simulink model "PMSM_FOC_sensorless"  (R2026a)
settings: Solver=FixedStepDiscrete  StopTime=10  FixedStep=Ts  EnableMultiTasking=on
InitFcn:
  | ParameterInit
undefined symbols (not defined in the file): drive, FAKF, motor, Ts
libraries: simulink x10, mcbhdlcontrolslib x10, matrix_library x8, mcbcontrolslib x6, mcbpositiondecoderlib x3, mcbsensorlessestimatorlib x2, mcbeeMathTransformLib x2, slpidlib x2, sl_discontinuities x1, mcbplantlib x1, autolibpmsminterior x1, realtime_pacer_lib x1
(part 1 of 3)
settings Model: SimulationMode=accelerator  SnapshotBufferSize=100  Creator=xueji  LastModifiedBy=xuejf
settings DataIOCC: SaveFormat=StructureWithTime
settings OptimizationCC: ConditionallyExecuteInputs=off  UseDivisionForNetSlopeComputation=on  GainParamInheritBuiltInType=on  UseFloatMulNetSlope=on  StrengthReduction=on  NoFixptDivByZeroProtection=on  EfficientFloat2IntCast=on  OptimizationPriority=Speed  MultiThreadedLoops=on  AutoScheduleForLoops=on  UseRestrictQualifier=on
settings DebuggingCC: ParameterOverflowMsg=none  ParameterUnderflowMsg=error  ParameterPrecisionLossMsg=none
settings HardwareCC: ProdLargestAtomicInteger=Long  ProdLargestAtomicFloat=Double  ProdHWDeviceType=ARM Compatible->ARM Cortex  TargetBitPerPointer=64.0  TargetBitPerSizeT=64.0  TargetBitPerPtrDiffT=64.0  TargetLongLongMode=on  TargetIntDivRoundTo=Zero  TargetEndianess=LittleEndian  TargetWordSize=64.0  TargetHWDeviceType=MATLAB Host  ProdEqTarget=off
settings SFSimCC: SimTargetLang=C++
settings RTWCC: SystemTargetFile=ert.tlc  GenCodeOnly=on  Toolchain=GNU Tools for ARM Embedded Processors  BuildConfiguration=Faster Runs  DataTypeReplacement=CDataTypesFixedWidth  Description=Embedded Coder
settings CodeAppCC: CustomSymbolStrGlobalVar=rt$N$M  CustomSymbolStrType=$N$M  CustomSymbolStrFcn=$N$M$F  CustomSymbolStrMacro=$N$M  UseSimReservedNames=on
settings ERTTargetCC: ExtModeTransport=1.0  ExtModeMexFile=ext_serial_win32_comm  RootIOFormat=Structure reference  ERTFilePackagingFormat=Compact  IndentSize=4  MaxIdInt64=INT64_MAX  MinIdInt64=INT64_MIN  MaxIdUint64=UINT64_MAX  MaxIdInt32=INT32_MAX  MinIdInt32=INT32_MIN  MaxIdUint32=UINT32_MAX  MaxIdInt16=INT16_MAX  MinIdInt16=INT16_MIN  MaxIdUint16=UINT16_MAX  MaxIdInt8=INT8_MAX  MinIdInt8=INT8_MIN  MaxIdUint8=UINT8_MAX  DynamicArrayContainerType=coder::array  SupportAbsoluteTime=off  CodeInterfacePackaging=Reusable function  SupportComplex=off
settings SimscapeCC: SimscapeNominalValues="[{\"value\":\"1\",\"unit\":\"A\"},{\"value\":\"1\",\"unit\":\"bar\"},{\"value\":\"1\",\"unit\":\"cm^2\"},{\"value\":\"1\",\"unit\":\"cm^3/s\"},{\"value\":\"1\",\"unit\":\"kJ/kg\"},{\"value\":\"1\",\"unit\":\"kW\"},{\"value\":\"1\",\"unit\":\"l\"},{\"value\":\"1\",\"unit\":\"N\"},{\"value\":\"1\",\"unit\":\"N*m\"},{\"value\":\"1\",\"unit\":\"V\"}]"  SimscapeLogType=none  SimscapeLogDataHistory=5000.0

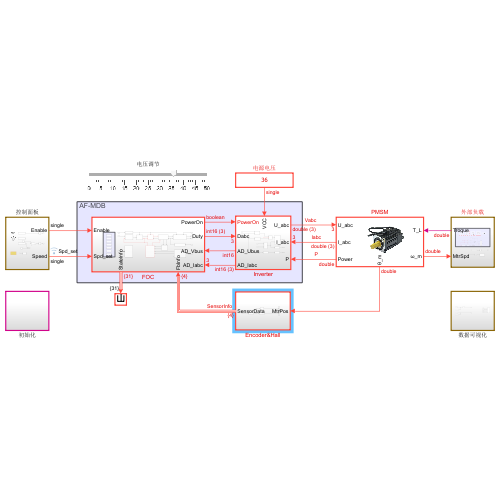
[thumbnail: Simulink's stored preview of the top-level diagram]
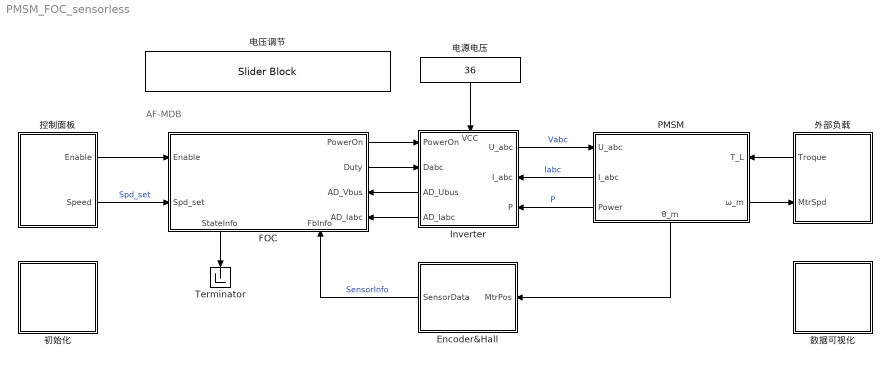
== system PMSM_FOC_sensorless ==
  note: AF-MDB
  Encoder&Hall : Subsystem
      settings: PortSchema="{\"entries\":[{\"content\":{\"sides\":[{\"content\":{\"connectorIds\":[\"Out1\"]},\"type\":\"ConnectorPlacement.EquallySpacedRectSide\",\"uuid\":\"8fa3dea7-ffc3-491e-9276-c955a36c6f18\"},{\"content\":{\"connectorIds\":[\"In1\"],\"side\":\"RIGHT\"},\"type\":\"ConnectorPlacement.EquallySpacedRectSide\",\"uuid\":\"8834e5d4-3827-462b-95b1-89ca8135bf93\"},{\"content\":{\"connectorIds\":[],\"side\":\"TOP\"},\"type\":\"ConnectorPlacement.EquallySpacedRectSide\",\"uuid\":\"076dd7d4-9aaa-4226-b42d-66fe25b6b28f\"}]},\"type\":\"ConnectorPlacement.EquallySpacedConnector\",\"uuid\":\"9a578460-81ff-4443-b5ec-3bd826764958\"}],\"packageUris\":[\"http://schema.mathworks.com/mf0/Connector/R2020b\"],\"version\":\"1.0\"}"
  FOC : Subsystem
      settings: PortSchema="{\"entries\":[{\"content\":{\"sides\":[{\"content\":{\"connectorIds\":[\"In1\",\"In2\"]},\"type\":\"ConnectorPlacement.EquallySpacedRectSide\",\"uuid\":\"46e73fc8-9e26-46f5-900f-d300c3d3ffa4\"},{\"content\":{\"connectorIds\":[\"Out1\",\"Out2\",\"In4\",\"In5\"],\"side\":\"RIGHT\"},\"type\":\"ConnectorPlacement.EquallySpacedRectSide\",\"uuid\":\"f8f13760-52ab-4821-8986-2e35fedfc95a\"},{\"content\":{\"side\":\"TOP\"},\"type\":\"ConnectorPlacement.EquallySpacedRectSide\",\"uuid\":\"3755d0d3-c979-48bd-b55d-3cbbf7594976\"},{\"content\":{\"connectorIds\":[\"Out3\",\"In3\"],\"side\":\"BOTTOM\"},\"type\":\"ConnectorPlacement.EquallySpacedRectSide\",\"uuid\":\"2c00eda5-e8e0-415c-bf0a-f2eb27cf355a\"}]},\"type\":\"ConnectorPlacement.EquallySpacedConnector\",\"uuid\":\"0d2281d8-e320-4044-ba1a-0a9e2c9cef92\"}],\"packageUris\":[\"http://schema.mathworks.com/mf0/Connector/R2020b\"],\"version\":\"1.0\"}"
  Inverter : Subsystem
      settings: PortSchema="{\"entries\":[{\"content\":{\"sides\":[{\"content\":{\"connectorIds\":[\"In1\",\"In2\",\"Out2\",\"Out3\"]},\"type\":\"ConnectorPlacement.EquallySpacedRectSide\",\"uuid\":\"edbc1bf3-6f5f-4012-892f-584587f9ac82\"},{\"content\":{\"connectorIds\":[\"Out1\",\"In4\",\"In5\"],\"side\":\"RIGHT\"},\"type\":\"ConnectorPlacement.EquallySpacedRectSide\",\"uuid\":\"6f51a7d6-6c28-4294-91cd-551043c21fcb\"},{\"content\":{\"connectorIds\":[\"In3\"],\"side\":\"TOP\"},\"type\":\"ConnectorPlacement.EquallySpacedRectSide\",\"uuid\":\"ca45aa73-ffa8-42f2-be70-f61dd7061c22\"}]},\"type\":\"ConnectorPlacement.EquallySpacedConnector\",\"uuid\":\"c09c89a4-9801-4f10-8b25-4ff06a898cdd\"}],\"packageUris\":[\"http://schema.mathworks.com/mf0/Connector/R2020b\"],\"version\":\"1.0\"}"
  PMSM : Subsystem
      settings: PortSchema="{\"entries\":[{\"content\":{\"sides\":[{\"content\":{\"connectorIds\":[\"In1\",\"Out3\",\"Out4\"]},\"type\":\"ConnectorPlacement.EquallySpacedRectSide\",\"uuid\":\"c2b23440-fc85-4d9c-858e-b988650f87d0\"},{\"content\":{\"connectorIds\":[\"In2\",\"Out1\"],\"side\":\"RIGHT\"},\"type\":\"ConnectorPlacement.EquallySpacedRectSide\",\"uuid\":\"6d28ba24-87ca-4dc4-bb5b-31bd216445dc\"},{\"content\":{\"side\":\"TOP\"},\"type\":\"ConnectorPlacement.EquallySpacedRectSide\",\"uuid\":\"4591baad-8ef3-475b-84da-7f88249a3560\"},{\"content\":{\"connectorIds\":[\"Out2\"],\"side\":\"BOTTOM\"},\"type\":\"ConnectorPlacement.EquallySpacedRectSide\",\"uuid\":\"01b968b1-c8c0-4355-9518-8898278f5093\"}]},\"type\":\"ConnectorPlacement.EquallySpacedConnector\",\"uuid\":\"f1130276-be58-456e-bfcb-28f536690efa\"}],\"packageUris\":[\"http://schema.mathworks.com/mf0/Connector/R2020b\"],\"version\":\"1.0\"}"
      mask Display: image('$imagefile'); % 使用工具条上的 "编辑图像" 进行更改。
  Terminator : Terminator
  初始化 : Subsystem
  外部负载 : Subsystem
      settings: PortSchema="{\"entries\":[{\"content\":{\"sides\":[{\"content\":{\"connectorIds\":[]},\"type\":\"ConnectorPlacement.EquallySpacedRectSide\",\"uuid\":\"5c626d5b-bf7f-42ce-ab58-2d542e2344bf\"},{\"content\":{\"connectorIds\":[\"Out1\",\"In1\"],\"side\":\"RIGHT\"},\"type\":\"ConnectorPlacement.EquallySpacedRectSide\",\"uuid\":\"d15cb2d3-f4cc-4d71-a0ed-13294ce13e05\"},{\"content\":{\"connectorIds\":[],\"side\":\"TOP\"},\"type\":\"ConnectorPlacement.EquallySpacedRectSide\",\"uuid\":\"7acbd73b-52e8-4e77-ba06-f51650d8c153\"}]},\"type\":\"ConnectorPlacement.EquallySpacedConnector\",\"uuid\":\"b6d8bd3c-2124-439b-8d25-1ae7167828cc\"}],\"packageUris\":[\"http://schema.mathworks.com/mf0/Connector/R2020b\"],\"version\":\"1.0\"}"
  控制面板 : Subsystem
  数据可视化 : Subsystem
  电压调节 : SliderBlock  LabelPosition=Hide  ScaleMax=50  TickInterval=5
  电源电压 : Constant  Value=36  OutDataTypeStr=single  SampleTime=Ts
  wires:
  Inverter/1(U_abc) -> PMSM/1(U_abc)  "Vabc"
  电源电压/1 -> Inverter/3(VCC)
  FOC/2(Duty) -> Inverter/2(Dabc)
  控制面板/1(Enable) -> FOC/1(Enable)
  控制面板/2(Speed) -> FOC/2(Spd_set)  "Spd_set"
  外部负载/1(Troque) -> PMSM/2(T_L)
  PMSM/1(ω_m) -> 外部负载/1(MtrSpd)
  PMSM/3(I_abc) -> Inverter/4(I_abc)  "Iabc"
  Inverter/2(AD_Ubus) -> FOC/4(AD_Vbus)
  FOC/3(StateInfo) -> Terminator/1
  FOC/1(PowerOn) -> Inverter/1(PowerOn)
  Inverter/3(AD_Iabc) -> FOC/5(AD_Iabc)
  PMSM/4(Power) -> Inverter/5(P)  "P"
  PMSM/2(θ_m) -> Encoder&Hall/1(MtrPos)
  Encoder&Hall/1(SensorData) -> FOC/3(FbInfo)  "SensorInfo"

== system PMSM_FOC_sensorless/Encoder&Hall ==
  MtrPos : Inport
  Bus Creator : BusCreator  Inputs=2
  Data Type Conversion3 : DataTypeConversion  OutDataTypeStr=single  SaturateOnIntegerOverflow=off  RndMeth=Floor
  编码器 : Subsystem
  霍尔传感器 : Subsystem
  SensorData : Outport
  wires:
  Bus Creator/1 -> SensorData/1
  编码器/1(编码值) -> Bus Creator/2  "Encoder"
  MtrPos/1 -> Data Type Conversion3/1
  Data Type Conversion3/1 -> 编码器/1(<MtrPos>), 霍尔传感器/1(MtrPos)  "MtrPos"
  霍尔传感器/1(Hall) -> Bus Creator/1  "Hall"

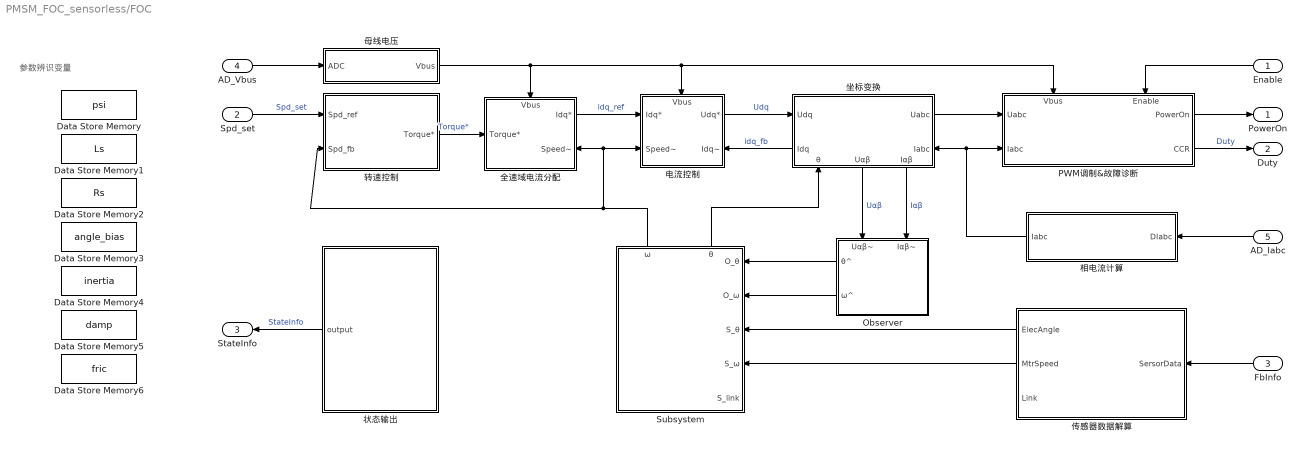
== system PMSM_FOC_sensorless/FOC ==
  note: 参数辨识变量
  Enable : Inport
  Spd_set : Inport  Port=2
  FbInfo : Inport  Port=3
  AD_Vbus : Inport  Port=4
  AD_Iabc : Inport  Port=5
  Data Store Memory : DataStoreMemory  DataStoreName=psi  WriteAfterWriteMsg=warning  ShowAdditionalParam=off
  Data Store Memory1 : DataStoreMemory  DataStoreName=Ls  WriteAfterWriteMsg=warning  ShowAdditionalParam=off
  Data Store Memory2 : DataStoreMemory  DataStoreName=Rs  WriteAfterWriteMsg=warning  ShowAdditionalParam=off
  Data Store Memory3 : DataStoreMemory  DataStoreName=angle_bias  WriteAfterWriteMsg=warning  ShowAdditionalParam=off  OutDataTypeStr=single
  Data Store Memory4 : DataStoreMemory  DataStoreName=inertia  WriteAfterWriteMsg=warning  ShowAdditionalParam=off  OutDataTypeStr=single
  Data Store Memory5 : DataStoreMemory  DataStoreName=damp  WriteAfterWriteMsg=warning  ShowAdditionalParam=off  OutDataTypeStr=single
  Data Store Memory6 : DataStoreMemory  DataStoreName=fric  WriteAfterWriteMsg=warning  ShowAdditionalParam=off  OutDataTypeStr=single
  Observer : Subsystem
      settings: MinAlgLoopOccurrences=on  PortSchema="{\"entries\":[{\"content\":{\"sides\":[{\"content\":{\"connectorIds\":[\"Out1\",\"Out2\"]},\"type\":\"ConnectorPlacement.EquallySpacedRectSide\",\"uuid\":\"e0bc5786-ce1d-4855-a3b5-736cd4452aa5\"},{\"content\":{\"side\":\"RIGHT\"},\"type\":\"ConnectorPlacement.EquallySpacedRectSide\",\"uuid\":\"2fd42ec2-cdfa-4ba6-bbae-150322a5d493\"},{\"content\":{\"connectorIds\":[\"In1\",\"In2\"],\"side\":\"TOP\"},\"type\":\"ConnectorPlacement.EquallySpacedRectSide\",\"uuid\":\"b90c8681-3a82-4d31-b956-3e10c61bd992\"}]},\"type\":\"ConnectorPlacement.EquallySpacedConnector\",\"uuid\":\"5605c3b5-9268-4421-a61a-19e31e78b2b2\"}],\"packageUris\":[\"http://schema.mathworks.com/mf0/Connector/R2020b\"],\"version\":\"1.0\"}"
  PWM调制&故障诊断 : Subsystem
      settings: PortSchema="{\"entries\":[{\"content\":{\"sides\":[{\"content\":{\"connectorIds\":[\"In1\",\"In2\"]},\"type\":\"ConnectorPlacement.EquallySpacedRectSide\",\"uuid\":\"492d6452-e717-42c4-995f-3faa38429cae\"},{\"content\":{\"connectorIds\":[\"Out1\",\"Out2\"],\"side\":\"RIGHT\"},\"type\":\"ConnectorPlacement.EquallySpacedRectSide\",\"uuid\":\"a45b9f70-76fb-43db-a233-80127821733d\"},{\"content\":{\"connectorIds\":[\"In3\",\"In4\"],\"side\":\"TOP\"},\"type\":\"ConnectorPlacement.EquallySpacedRectSide\",\"uuid\":\"87480e42-0fd9-4078-9596-9cf4a8d8a61b\"},{\"content\":{\"side\":\"BOTTOM\"},\"type\":\"ConnectorPlacement.EquallySpacedRectSide\",\"uuid\":\"e85548a5-948a-4384-9ce6-748091ec18d7\"}]},\"type\":\"ConnectorPlacement.EquallySpacedConnector\",\"uuid\":\"18d7a9be-c392-4737-8548-f782ad0f8f26\"}],\"packageUris\":[\"http://schema.mathworks.com/mf0/Connector/R2020b\"],\"version\":\"1.0\"}"
  Subsystem : Subsystem
      settings: PortSchema="{\"entries\":[{\"content\":{\"sides\":[{\"content\":{},\"type\":\"ConnectorPlacement.EquallySpacedRectSide\",\"uuid\":\"d4a4fcc6-9eab-45aa-b231-b7af833cd8c6\"},{\"content\":{\"connectorIds\":[\"In1\",\"In2\",\"In3\",\"In4\",\"In5\"],\"side\":\"RIGHT\"},\"type\":\"ConnectorPlacement.EquallySpacedRectSide\",\"uuid\":\"bf374db6-391b-4179-b18d-5bc8f845fc33\"},{\"content\":{\"connectorIds\":[\"Out1\",\"Out2\"],\"side\":\"TOP\"},\"type\":\"ConnectorPlacement.EquallySpacedRectSide\",\"uuid\":\"b7b6826e-7c33-41ba-b3c7-d16a7d7beb3a\"}]},\"type\":\"ConnectorPlacement.EquallySpacedConnector\",\"uuid\":\"61c6cbd8-a55e-4c51-8b84-52df934ee1be\"}],\"packageUris\":[\"http://schema.mathworks.com/mf0/Connector/R2020b\"],\"version\":\"1.0\"}"
  传感器数据解算 : Subsystem
  全速域电流分配 : Subsystem
      settings: PortSchema="{\"entries\":[{\"content\":{\"sides\":[{\"content\":{\"connectorIds\":[\"In1\"]},\"type\":\"ConnectorPlacement.EquallySpacedRectSide\",\"uuid\":\"55c1d0af-1e12-4135-aa70-ca0befd6bb29\"},{\"content\":{\"connectorIds\":[\"Out1\",\"In3\"],\"side\":\"RIGHT\"},\"type\":\"ConnectorPlacement.EquallySpacedRectSide\",\"uuid\":\"d5856c39-d2d9-42bf-88a6-12c62f6eb837\"},{\"content\":{\"connectorIds\":[\"In2\"],\"side\":\"TOP\"},\"type\":\"ConnectorPlacement.EquallySpacedRectSide\",\"uuid\":\"f04465a3-695d-494e-bf21-7b8ba0e1a298\"}]},\"type\":\"ConnectorPlacement.EquallySpacedConnector\",\"uuid\":\"e6412d78-9d8b-45ef-81b3-23a4fb87ae10\"}],\"packageUris\":[\"http://schema.mathworks.com/mf0/Connector/R2020b\"],\"version\":\"1.0\"}"
  坐标变换 : Subsystem
      settings: PortSchema="{\"entries\":[{\"content\":{\"sides\":[{\"content\":{\"connectorIds\":[\"In1\",\"Out4\"]},\"type\":\"ConnectorPlacement.EquallySpacedRectSide\",\"uuid\":\"19423b74-9855-4da1-a32f-fc09d117de38\"},{\"content\":{\"connectorIds\":[\"Out1\",\"In3\"],\"side\":\"RIGHT\"},\"type\":\"ConnectorPlacement.EquallySpacedRectSide\",\"uuid\":\"45d897d7-b2dc-4681-bc4b-90a4bd929118\"},{\"content\":{\"connectorIds\":[],\"side\":\"TOP\"},\"type\":\"ConnectorPlacement.EquallySpacedRectSide\",\"uuid\":\"59354a96-0169-49af-a302-86e785c620a3\"},{\"content\":{\"connectorIds\":[\"In2\",\"Out2\",\"Out3\"],\"side\":\"BOTTOM\"},\"type\":\"ConnectorPlacement.EquallySpacedRectSide\",\"uuid\":\"fb332ee8-d153-4216-8303-19cfa3862110\"}]},\"type\":\"ConnectorPlacement.EquallySpacedConnector\",\"uuid\":\"5f6d72a6-e6b8-48f2-bb88-1ad3720f15b2\"}],\"packageUris\":[\"http://schema.mathworks.com/mf0/Connector/R2020b\"],\"version\":\"1.0\"}"
  母线电压 : Subsystem
  状态输出 : Subsystem
      settings: PortSchema="{\"entries\":[{\"content\":{\"sides\":[{\"content\":{\"connectorIds\":[\"Out1\"]},\"type\":\"ConnectorPlacement.EquallySpacedRectSide\",\"uuid\":\"5ecb5947-9baa-4bfe-8641-96ff20667d62\"},{\"content\":{\"side\":\"RIGHT\"},\"type\":\"ConnectorPlacement.EquallySpacedRectSide\",\"uuid\":\"3d186154-f081-4d30-a108-1a942147f536\"},{\"content\":{\"side\":\"TOP\"},\"type\":\"ConnectorPlacement.EquallySpacedRectSide\",\"uuid\":\"5aa511f5-28fe-4d78-8a7e-f2efec5693a1\"}]},\"type\":\"ConnectorPlacement.EquallySpacedConnector\",\"uuid\":\"ee06c015-bb25-435b-b725-56d91e20a522\"}],\"packageUris\":[\"http://schema.mathworks.com/mf0/Connector/R2020b\"],\"version\":\"1.0\"}"
  电流控制 : Subsystem
      settings: PortSchema="{\"entries\":[{\"content\":{\"sides\":[{\"content\":{\"connectorIds\":[\"In1\",\"In2\"]},\"type\":\"ConnectorPlacement.EquallySpacedRectSide\",\"uuid\":\"bf76b923-f33f-405a-8981-aa5371d2085f\"},{\"content\":{\"connectorIds\":[\"Out1\",\"In4\"],\"side\":\"RIGHT\"},\"type\":\"ConnectorPlacement.EquallySpacedRectSide\",\"uuid\":\"e7d4bdbe-138f-4605-8031-f7f1fbb983cf\"},{\"content\":{\"connectorIds\":[\"In3\"],\"side\":\"TOP\"},\"type\":\"ConnectorPlacement.EquallySpacedRectSide\",\"uuid\":\"9cdf7367-4fd9-4634-a6c3-b049cc73c34c\"},{\"content\":{\"side\":\"BOTTOM\"},\"type\":\"ConnectorPlacement.EquallySpacedRectSide\",\"uuid\":\"aba65895-d8a9-40f0-9a72-aa89d29f659a\"}]},\"type\":\"ConnectorPlacement.EquallySpacedConnector\",\"uuid\":\"3c2b3690-9a24-4e84-8e12-40b94ce0a856\"}],\"packageUris\":[\"http://schema.mathworks.com/mf0/Connector/R2020b\"],\"version\":\"1.0\"}"
  相电流计算 : Subsystem
  转速控制 : Subsystem
  PowerOn : Outport
  Duty : Outport  Port=2
  StateInfo : Outport  Port=3
  wires:
  PWM调制&故障诊断/2(CCR) -> Duty/1  "Duty"
  坐标变换/4(Idq) -> 电流控制/4(Idq~)  "idq_fb"
  电流控制/1(Udq*) -> 坐标变换/1(Udq)  "Udq"
  坐标变换/1(Uabc) -> PWM调制&故障诊断/1(Uabc)
  Enable/1 -> PWM调制&故障诊断/4(Enable)
  坐标变换/2(Uαβ) -> Observer/1(Uαβ~)  "Uαβ"
  坐标变换/3(Iαβ) -> Observer/2(Iαβ~)  "Iαβ"
  Spd_set/1 -> 转速控制/1(Spd_ref)  "Spd_set"
  转速控制/1(Torque*) -> 全速域电流分配/1(Torque*)  "Torque*"
  全速域电流分配/1(Idq*) -> 电流控制/1(Idq*)  "idq_ref"
  相电流计算/1(Iabc) -> 坐标变换/3(Iabc), PWM调制&故障诊断/2(Iabc)
  FbInfo/1 -> 传感器数据解算/1(SersorData)
  状态输出/1(output) -> StateInfo/1  "StateInfo"
  PWM调制&故障诊断/1(PowerOn) -> PowerOn/1
  AD_Iabc/1 -> 相电流计算/1(DIabc)
  母线电压/1(Vbus) -> PWM调制&故障诊断/3(Vbus), 电流控制/3(Vbus), 全速域电流分配/2(Vbus)
  AD_Vbus/1 -> 母线电压/1(ADC)
  传感器数据解算/2(MtrSpeed) -> Subsystem/4(S_ω)
  传感器数据解算/1(ElecAngle) -> Subsystem/3(S_θ)
  Subsystem/1(ω) -> 电流控制/2(Speed~), 全速域电流分配/3(Speed~), 转速控制/2(Spd_fb)
  Observer/1(θ^) -> Subsystem/1(O_θ)
  Subsystem/2(θ) -> 坐标变换/2(θ)
  Observer/2(ω^) -> Subsystem/2(O_ω)

== system PMSM_FOC_sensorless/Inverter ==
  PowerOn : Inport
  Dabc : Inport  Port=2
  VCC : Inport  Port=3
  I_abc : Inport  Port=4
  P : Inport  Port=5
  AD转换 : Subsystem
  Data Type Conversion1 : DataTypeConversion  OutDataTypeStr=single  SaturateOnIntegerOverflow=off  RndMeth=Floor
  Switch : Switch  Criteria=u2 > Threshold  SaturateOnIntegerOverflow=off  InputSameDT=off
  模拟MOS管截至状态 : Subsystem  TreatAsAtomicUnit=on
  正常PWM调制 : Subsystem  TreatAsAtomicUnit=on
  母线压降 : Subsystem
  母线电压采样 : Subsystem
  逆变器 : mcbplantlib/Average-Value Inverter
  采样芯片 : Subsystem
  U_abc : Outport
  AD_Ubus : Outport  Port=2
  AD_Iabc : Outport  Port=3
  wires:
  逆变器/1 -> U_abc/1
  PowerOn/1 -> Switch/2
  模拟MOS管截至状态/1(Out1) -> Switch/3
  正常PWM调制/1(Out1) -> Switch/1
  Switch/1 -> 逆变器/1
  Dabc/1 -> 正常PWM调制/1(Dabc)
  Data Type Conversion1/1 -> 采样芯片/1(Iabc)  "Iabc"
  I_abc/1 -> Data Type Conversion1/1, 模拟MOS管截至状态/1(Iabc), 正常PWM调制/2(Iabc)
  AD转换/1(digital) -> AD_Iabc/1  "ADC_Iabc"
  采样芯片/1(Isabc) -> AD转换/1(analog)
  母线电压采样/1(AD_Ubus) -> AD_Ubus/1
  P/1 -> 母线压降/2(P)
  母线压降/1(U_bus) -> 母线电压采样/1(U_bus), 逆变器/2
  VCC/1 -> 母线压降/1(VCC)

== system PMSM_FOC_sensorless/PMSM ==
  U_abc : Inport
  T_L : Inport  Port=2
  Bus Selector : BusSelector  OutputSignals=PwrInfo.PwrTrnsfrd.PwrBus,MtrPos
  Interior PMSM : autolibpmsminterior/Interior PMSM  port_config=Torque  sim_type=Discrete  Ts=Ts  FilePath=interiorpmsm_motordata.m  P=motor.P  Rs=motor.Rs  Ldq=[motor.Ls motor.Ls]  KConstText=Back-emf constant (Ke):  lambda_pm=0.1194  Ke=motor.Ke  mechanical=[motor.J, motor.damp, motor.fric]  idq0=[0 0]  theta_init=motor.angle_init  omega_init=0  KConst=motor.Ke  lambda_pm_calc=0.010526  Kt=1.323  RefBlkName='autolibpmsminterior/Interior PMSM'  aMode=1
      settings: LibrarySourceBlock=autolibemachines/Interior PMSM
  Mechanical to Electrical Position : mcbpositiondecoderlib/Mechanical to Electrical Position  PolePairsInputType=Specify via dialog  NrPP=motor.P  selectedRange=Radians  MechOfstInputType=Specify via dialog  mechOffsetIn=0  maxAngleIn=2*pi  InputDataType=single  VariantSelect=floating-point
      settings: LibrarySourceBlock=mcblib/Sensor Decoders/Mechanical to Electrical Position
  Subsystem2 : Subsystem
  ω_m : Outport
  θ_m : Outport  Port=2
  I_abc : Outport  Port=3
  Power : Outport  Port=4
  tag scope: Real_Iabc=global, Real_LdTrq=global, Real_MotorInfo=global, Real_MtrSpd=global, Real_Theat_e=global, Real_Theat_m=global, Real_Vabc=global
  wires:
  T_L/1 -> [Real_LdTrq], Interior PMSM/1
  Interior PMSM/3 -> [Real_MtrSpd], ω_m/1  "ω_m"
  Interior PMSM/2 -> [Real_Iabc], I_abc/1
  Interior PMSM/1 -> [Real_MotorInfo], Bus Selector/1  "MotorInfo"
  U_abc/1 -> [Real_Vabc], Interior PMSM/2
  Bus Selector/2 -> Mechanical to Electrical Position/1, [Real_Theat_m], θ_m/1  "<MtrPos>"
  Bus Selector/1 -> Power/1  "<PwrBus>"
  Mechanical to Electrical Position/1 -> Subsystem2/1(0-2pi)
  Subsystem2/1(-pi-pi) -> [Real_Theat_e]  "θ_e"

== system PMSM_FOC_sensorless/初始化 ==

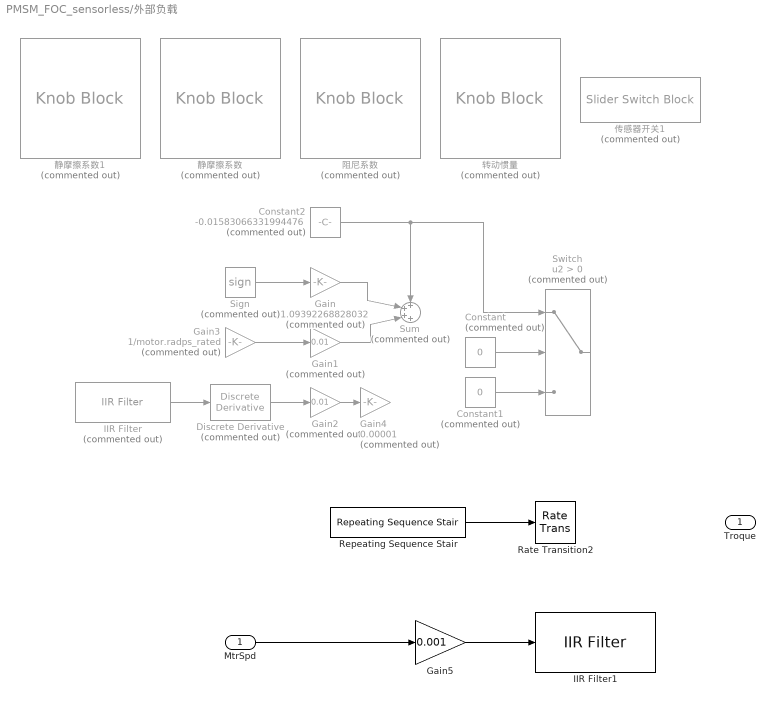
== system PMSM_FOC_sensorless/外部负载 ==
  MtrSpd : Inport
  Constant : Constant  Commented=on  Value=0
  Constant1 : Constant  Commented=on  Value=0
  Constant2 : Constant  Commented=on  Value=-0.01583066331994476
  Discrete Derivative : simulink/Discrete/Discrete Derivative  Commented=on  gainval=1.0  ICPrevScaledInput=0.0  OutMin=[]  OutMax=[]  OutDataType=fixdt(1, 16)  OutScaling=2^-10  DoSatur=off
  Gain : Gain  Commented=on  Gain=1.09392268828032
  Gain1 : Gain  Commented=on  Gain=0.01
  Gain2 : Gain  Commented=on  Gain=0.01
  Gain3 : Gain  Commented=on  Gain=1/motor.radps_rated
  Gain4 : Gain  Commented=on  Gain=0.00001
  Gain5 : Gain  Gain=0.001
  IIR Filter : mcbcontrolslib/IIR Filter  Commented=on  VariantControl=Low Pass Filter  VariantSelect=Low-pass  FilterConstantInputType=Specify via dialog  Filter_constant=0.1  advancedSettings=off  Ts=50e-6  cutOff_freq=353.6777
      settings: LibrarySourceBlock=mcbhdllib/Signal Management/IIR Filter
  IIR Filter1 : mcbhdlcontrolslib/IIR Filter  VariantControl=Low Pass Filter  VariantSelect=Low-pass  FilterConstantInputType=Specify via dialog  Filter_constant=0.01  advancedSettings=off  Ts=50e-6  cutOff_freq=32.1525
  Rate Transition2 : RateTransition  OutPortSampleTime=Ts
  Repeating Sequence Stair : simulink/Sources/Repeating Sequence Stair  OutValues=0.3*[0 0 0 motor.T_rated motor.T_rated motor.T_rated 0 0 0].'  tsamp=0.5  OutMin=[]  OutMax=[]  OutDataTypeStr=double  OutputDataTypeScalingMode=double  OutDataType=fixdt(0,8)  ConRadixGroup=Best Precision: Vector-wise  OutScaling=2^-12
  Sign : Signum  Commented=on
  Sum : Sum  Commented=on  Inputs=++++
  Switch : Switch  Commented=on  Criteria=u2 > Threshold  SaturateOnIntegerOverflow=off  InputSameDT=off
  传感器开关1 : SliderSwitchBlock  Commented=on
  转动惯量 : KnobBlock  Commented=on  ScaleMin=0.01  ScaleType=Log
  阻尼系数 : KnobBlock  Commented=on  ScaleMin=0.01  ScaleType=Log
  静摩擦系数 : KnobBlock  Commented=on  ScaleMin=0.01  ScaleType=Log
  静摩擦系数1 : KnobBlock  Commented=on  ScaleMin=-1  ScaleMax=1
  Troque : Outport
  wires:
  ? -> Sign/1, IIR Filter/1, Gain3/1
  Sign/1 -> Gain/1
  Gain/1 -> Sum/2
  Constant2/1 -> Switch/1, Sum/1
  Constant/1 -> Switch/2
  Constant1/1 -> Switch/3
  Discrete Derivative/1 -> Gain2/1
  Gain1/1 -> Sum/3
  Gain3/1 -> Gain1/1
  Gain2/1 -> Gain4/1
  IIR Filter/1 -> Discrete Derivative/1
  Repeating Sequence Stair/1 -> Rate Transition2/1
  MtrSpd/1 -> Gain5/1
  Gain5/1 -> IIR Filter1/1

== system PMSM_FOC_sensorless/控制面板 ==
  Clock : Clock
  Constant3 : Constant  OutDataTypeStr=single  SampleTime=Ts
  Gain3 : Gain  Gain=motor.radps_rated  OutDataTypeStr=single
  Knob : KnobBlock  ScaleMin=-1  ScaleMax=1
  MATLAB Function : MATLAB Function  TreatAsAtomicUnit=on
  Product : Product
  Rate Transition2 : RateTransition  OutPortSampleTime=Ts
  Rate Transition3 : RateTransition  OutPortSampleTime=Ts
  Real-Time Pacer : realtime_pacer_lib/Real-Time Pacer  Commented=on  simTimePerRealTime=0.1
      settings: SourceProductName=Real-Time Pacer
  Repeating Sequence Stair1 : simulink/Sources/Repeating Sequence Stair  OutValues=[0.05 -0.05 -1 1]  tsamp=0.5  OutMin=[]  OutMax=[]  OutDataTypeStr=double  OutputDataTypeScalingMode=double  OutDataType=fixdt(0,8)  ConRadixGroup=Best Precision: Vector-wise  OutScaling=2^-12
  Sine Wave : Sin  Amplitude=0.2  Bias=0.2  Frequency=2*pi  Phase=-pi/2  SampleTime=Ts
  Step : Step  SampleTime=0
  传感器开关 : SliderSwitchBlock
  可调 : Constant  Value=0.5764853922526041  OutDataTypeStr=single  SampleTime=Ts
  Enable : Outport
  Speed : Outport  Port=2
  wires:
  Gain3/1 -> Rate Transition2/1
  Constant3/1 -> Rate Transition3/1
  Rate Transition2/1 -> Speed/1
  Rate Transition3/1 -> Enable/1
  Sine Wave/1 -> Product/1
  Step/1 -> Product/2
  Repeating Sequence Stair1/1 -> Gain3/1
  Clock/1 -> MATLAB Function/1(t)

== system PMSM_FOC_sensorless/数据可视化 ==
  Sum : Sum  Inputs=|+-
  Sum1 : Sum  Inputs=|+-
  Terminator : Terminator
  Terminator1 : Terminator
  angle limit2 : Subsystem
  卡尔曼过程可视化 : Subsystem  mask{en=0, plot_freq=2000, buff_len=64, range=30}
      mask prompts: en "使能"; plot_freq "绘图频率"; buff_len "轨迹长度"; range "坐标范围"
      mask DialogControl DescGroupVar Prompt: 描述
      mask DialogControl DescTextVar Prompt: 卡尔曼观测器数据可视化
      mask DialogControl ParameterGroupVar Prompt: 参数
  wires:
  [x] -> 卡尔曼过程可视化/5(x_k)
  [x_1] -> 卡尔曼过程可视化/1(x_k|k-1)
  [P_1] -> 卡尔曼过程可视化/2(P_k|k-1)
  [z] -> 卡尔曼过程可视化/3(z_k)
  [R] -> 卡尔曼过程可视化/4(R)
  [P] -> 卡尔曼过程可视化/6(P_k)
  Sum/1 -> angle limit2/1(In)
  [Real_MtrSpd] -> Sum1/1
  angle limit2/1(Out) -> Terminator/1  "err_θ"
  Sum1/1 -> Terminator1/1  "err_ω"
  [Real_Theat_e] -> Sum/1
  [Observer_Speed_m] -> Sum1/2
  [Observer_Angle_e] -> Sum/2

== system PMSM_FOC_sensorless/Encoder&Hall/编码器 ==
  <MtrPos> : Inport
  Constant1 : Constant  Value=motor.ENC_CNT  OutDataTypeStr=int16
  Gain1 : Gain  Gain=motor.ENC_CNT/(2*pi)  OutDataTypeStr=int16
  Mod : Math  Operator=mod
  Sum : Sum  Inputs=|+-
  初始角度 : Constant  Value=motor.angle_init  OutDataTypeStr=single
  编码值 : Outport
  wires:
  <MtrPos>/1 -> Sum/1
  Sum/1 -> Gain1/1
  初始角度/1 -> Sum/2
  Constant1/1 -> Mod/2
  Gain1/1 -> Mod/1
  Mod/1 -> 编码值/1

== system PMSM_FOC_sensorless/Encoder&Hall/霍尔传感器 ==
  MtrPos : Inport
  Constant18 : Constant  Value=[1,0,1]  OutDataTypeStr=int8
  Constant19 : Constant  Value=[1,0,0]  OutDataTypeStr=int8
  Constant20 : Constant  Value=[1,1,0]  OutDataTypeStr=int8
  Constant21 : Constant  Value=[0,1,0]  OutDataTypeStr=int8
  Constant22 : Constant  Value=[0,1,1]  OutDataTypeStr=int8
  Constant23 : Constant  Value=[0,0,1]  OutDataTypeStr=int8
  Multiport Switch3 : MultiPortSwitch  DataPortOrder=Zero-based contiguous  Inputs=6  zeroidx=on  SaturateOnIntegerOverflow=off  InputSameDT=off
  Subsystem : Subsystem
  Hall : Outport
  wires:
  MtrPos/1 -> Subsystem/1(MtrPos)
  Subsystem/1(Phase) -> Multiport Switch3/1
  Multiport Switch3/1 -> Hall/1
  Constant18/1 -> Multiport Switch3/2
  Constant19/1 -> Multiport Switch3/3
  Constant20/1 -> Multiport Switch3/4
  Constant21/1 -> Multiport Switch3/5
  Constant22/1 -> Multiport Switch3/6
  Constant23/1 -> Multiport Switch3/7

== system PMSM_FOC_sensorless/FOC/Observer ==
  Uαβ~ : Inport
  Iαβ~ : Inport  Port=2
  AKF : Subsystem
  Demux : Demux  Outputs=2
  位置提取 : Subsystem
  对比观测器 : Subsystem  Commented=on
  角度转换 : Subsystem
  计算转子反电动势 : Subsystem
  转矩计算 : Subsystem
  θ^ : Outport
  ω^ : Outport  Port=2
  tag scope: Observer_Angle_e=global, Observer_Speed_m=global
  wires:
  Demux/1 -> ω^/1, [Observer_Speed_m]
  角度转换/1(sincos) -> 转矩计算/1(θ_sincos), 位置提取/2(θ_sincos)
  Uαβ~/1 -> 计算转子反电动势/2(Uαβ), 对比观测器/1(u)
  计算转子反电动势/1(Eαβ) -> 位置提取/1(Eαβ)  "E_αβ"
  Iαβ~/1 -> 计算转子反电动势/1(Iαβ), 转矩计算/2(I_αβ), 对比观测器/2(i)
  转矩计算/1(T) -> AKF/1(u_k)  "T"
  位置提取/1(ωθ) -> AKF/2(z_k)  "ωθ~"
  AKF/1(x_k) -> Demux/1
  Demux/2 -> [Observer_Angle_e], θ^/1, 角度转换/1(θ)

== system PMSM_FOC_sensorless/FOC/PWM调制&故障诊断 ==
  Uabc : Inport
  Iabc : Inport  Port=2
  Vbus : Inport  Port=3
  Enable : Inport  Port=4
  Constant : Constant  Value=0.5  OutDataTypeStr=single
  Divide : Product  Inputs=*/
  Gain1 : Gain  Gain=drive.dead_time/drive.T_PWM  OutDataTypeStr=single
  Gain3 : Gain  Gain=drive.CNT_PWM  OutDataTypeStr=int16
  NOT : Logic  Operator=NOT  IconShape=distinctive  AllPortsSameDT=off  OutDataTypeStr=boolean
  NOT1 : Logic  IconShape=distinctive  AllPortsSameDT=off  OutDataTypeStr=boolean
  Sign : Signum
  Sum : Sum  Inputs=+++
  故障诊断 : Subsystem
  限幅1 : Saturate  UpperLimit=drive.CNT_PWM*0.99  LowerLimit=drive.CNT_PWM*0.01
  PowerOn : Outport
  CCR : Outport  Port=2
  tag scope: U_bus=global
  wires:
  Divide/1 -> Sum/2  "Duty"
  Uabc/1 -> Divide/1
  限幅1/1 -> CCR/1
  Sign/1 -> Gain1/1
  Iabc/1 -> 故障诊断/1(I_abc), Sign/1
  Gain1/1 -> Sum/1
  NOT/1 -> NOT1/1
  Enable/1 -> NOT1/2
  故障诊断/1(Err_code) -> NOT/1
  NOT1/1 -> PowerOn/1
  Constant/1 -> Sum/3
  Sum/1 -> Gain3/1
  Vbus/1 -> [U_bus], Divide/2, 故障诊断/2(U_bus)
  Gain3/1 -> 限幅1/1

== system PMSM_FOC_sensorless/FOC/Subsystem ==
  O_θ : Inport
  O_ω : Inport  Port=2
  S_θ : Inport  Port=3
  S_ω : Inport  Port=4
  S_link : Inport  Port=5
  Switch : Switch  Criteria=u2 > Threshold  SaturateOnIntegerOverflow=off  InputSameDT=off
  Switch1 : Switch  Criteria=u2 > Threshold  SaturateOnIntegerOverflow=off  InputSameDT=off
  ω : Outport
  θ : Outport  Port=2
  wires:
  O_ω/1 -> Switch1/3
  S_θ/1 -> Switch/1
  O_θ/1 -> Switch/3
  S_ω/1 -> Switch1/1
  S_link/1 -> Switch1/2, Switch/2
  Switch/1 -> θ/1
  Switch1/1 -> ω/1

== system PMSM_FOC_sensorless/FOC/传感器数据解算 ==
  SersorData : Inport
  Bus Selector2 : BusSelector  OutputSignals=Hall,Encoder
  Terminator : Terminator
  角度计算 : Subsystem
  转速计算 : Subsystem
  ElecAngle : Outport
  MtrSpeed : Outport  Port=2
  Link : Outport  Port=3
  tag scope: Sensor_Angle_e=global, Sensor_Speed_m=global
  wires:
  SersorData/1 -> Bus Selector2/1
  角度计算/1(MtrPos) -> Terminator/1
  转速计算/1(MtrSpeed) -> [Sensor_Speed_m], MtrSpeed/1
  Bus Selector2/2 -> 转速计算/1(Encoder), 角度计算/2(Encoder)  "<Encoder>"
  Bus Selector2/1 -> 角度计算/1(Hall)  "<Hall>"
  角度计算/2(ElecAngle) -> [Sensor_Angle_e], ElecAngle/1
  角度计算/3(Link) -> Link/1

== system PMSM_FOC_sensorless/FOC/全速域电流分配 ==
  Torque* : Inport
  Vbus : Inport  Port=2
  Speed~ : Inport  Port=3
  Constant1 : Constant  Value=motor.I_max  OutDataTypeStr=single
  Gain : Gain  Gain=1/motor.Kt
  Gain2 : Gain  Gain=-1
  IIR Filter1 : mcbhdlcontrolslib/IIR Filter  VariantControl=Low Pass Filter  VariantSelect=Low-pass  FilterConstantInputType=Specify via dialog  Filter_constant=0.1  advancedSettings=off  Ts=50e-6  cutOff_freq=353.6777
  MJPA : Subsystem
  Math Function : Math  Operator=square
  Math Function1 : Math  Operator=square
  Mux1 : Mux  Inputs=2
  Saturation Dynamic : sl_discontinuities/Saturation Dynamic  OutMin=[]  OutMax=[]  OutDataTypeStr=single  OutDataType=fixdt(1, 16)  OutScaling=2^-10  DoSatur=off
  Sqrt : Sqrt
  Sum1 : Sum  Inputs=-+|
  Idq* : Outport
  tag scope: Speed_m=global
  wires:
  Saturation Dynamic/1 -> Mux1/2
  Mux1/1 -> IIR Filter1/1
  Torque*/1 -> Gain/1
  Speed~/1 -> MJPA/2(ω_m), [Speed_m]
  Constant1/1 -> Math Function1/1
  Math Function/1 -> Sum1/1
  Sum1/1 -> Sqrt/1
  Sqrt/1 -> Gain2/1, Saturation Dynamic/1
  Gain2/1 -> Saturation Dynamic/3
  Vbus/1 -> MJPA/1(Vbus)
  MJPA/1(i*_d) -> Math Function/1, Mux1/1
  Math Function1/1 -> Sum1/2
  IIR Filter1/1 -> Idq*/1
  Gain/1 -> Saturation Dynamic/2

== system PMSM_FOC_sensorless/FOC/坐标变换 ==
  Udq : Inport
  θ : Inport  Port=2
  Iabc : Inport  Port=3
  Subsystem11 : Subsystem
  Subsystem2 : Subsystem
      settings: PortSchema="{\"entries\":[{\"content\":{\"sides\":[{\"content\":{\"connectorIds\":[\"In1\"]},\"type\":\"ConnectorPlacement.EquallySpacedRectSide\",\"uuid\":\"492d6452-e717-42c4-995f-3faa38429cae\"},{\"content\":{\"connectorIds\":[\"Out1\"],\"side\":\"RIGHT\"},\"type\":\"ConnectorPlacement.EquallySpacedRectSide\",\"uuid\":\"a45b9f70-76fb-43db-a233-80127821733d\"},{\"content\":{\"connectorIds\":[\"In2\"],\"side\":\"TOP\"},\"type\":\"ConnectorPlacement.EquallySpacedRectSide\",\"uuid\":\"87480e42-0fd9-4078-9596-9cf4a8d8a61b\"},{\"content\":{\"connectorIds\":[],\"side\":\"BOTTOM\"},\"type\":\"ConnectorPlacement.EquallySpacedRectSide\",\"uuid\":\"abbb6dc7-6c8b-4aee-9a22-efe0eeab5972\"}]},\"type\":\"ConnectorPlacement.EquallySpacedConnector\",\"uuid\":\"18d7a9be-c392-4737-8548-f782ad0f8f26\"}],\"packageUris\":[\"http://schema.mathworks.com/mf0/Connector/R2020b\"],\"version\":\"1.0\"}"
  Subsystem3 : Subsystem
  Subsystem4 : Subsystem
  Subsystem5 : Subsystem
      settings: PortSchema="{\"entries\":[{\"content\":{\"sides\":[{\"content\":{\"connectorIds\":[\"In1\"]},\"type\":\"ConnectorPlacement.EquallySpacedRectSide\",\"uuid\":\"492d6452-e717-42c4-995f-3faa38429cae\"},{\"content\":{\"connectorIds\":[\"Out1\"],\"side\":\"RIGHT\"},\"type\":\"ConnectorPlacement.EquallySpacedRectSide\",\"uuid\":\"a45b9f70-76fb-43db-a233-80127821733d\"},{\"content\":{\"connectorIds\":[],\"side\":\"TOP\"},\"type\":\"ConnectorPlacement.EquallySpacedRectSide\",\"uuid\":\"87480e42-0fd9-4078-9596-9cf4a8d8a61b\"},{\"content\":{\"connectorIds\":[\"In2\"],\"side\":\"BOTTOM\"},\"type\":\"ConnectorPlacement.EquallySpacedRectSide\",\"uuid\":\"c5a9fd10-4005-478b-ab9c-ebed3c1e9985\"}]},\"type\":\"ConnectorPlacement.EquallySpacedConnector\",\"uuid\":\"18d7a9be-c392-4737-8548-f782ad0f8f26\"}],\"packageUris\":[\"http://schema.mathworks.com/mf0/Connector/R2020b\"],\"version\":\"1.0\"}"
  Uabc : Outport
  Uαβ : Outport  Port=2
  Iαβ : Outport  Port=3
  Idq : Outport  Port=4
  tag scope: I_abc=global, U_abc=global
  wires:
  Udq/1 -> Subsystem5/1(dq)
  Subsystem11/1(sincos) -> Subsystem2/2(sincos), Subsystem5/2(sincos)
  Subsystem5/1(αβ) -> Uαβ/1, Subsystem4/1(αβ)  "Uαβ"
  Subsystem3/1(αβ) -> Iαβ/1, Subsystem2/1(αβ)  "Iαβ"
  Subsystem2/1(dq) -> Idq/1  "Idq_fb"
  θ/1 -> Subsystem11/1(angle)  "E_angle"
  Subsystem4/1(abc) -> Uabc/1, [U_abc]
  Iabc/1 -> Subsystem3/1(abc), [I_abc]

== system PMSM_FOC_sensorless/FOC/母线电压 ==
  ADC : Inport
  Gain : Gain  Gain=drive.ADC_Vref/(drive.V_gain*drive.ADC_MaxCount*2)  OutDataTypeStr=single
  母线电压采样滤波 : mcbhdlcontrolslib/IIR Filter  VariantControl=Low Pass Filter  VariantSelect=Low-pass  FilterConstantInputType=Specify via dialog  Filter_constant=0.1  advancedSettings=off  Ts=50e-6  cutOff_freq=353.6777
  Vbus : Outport
  wires:
  Gain/1 -> 母线电压采样滤波/1
  母线电压采样滤波/1 -> Vbus/1
  ADC/1 -> Gain/1

== system PMSM_FOC_sensorless/FOC/状态输出 ==
  Bus Creator1 : BusCreator  Inputs=4
  Bus Creator2 : BusCreator  Inputs=4
  Bus Creator4 : BusCreator  Inputs=2
  Bus Creator6 : BusCreator  Inputs=7
  Constant : Constant  Value=0  OutDataTypeStr=single
  output : Outport
  wires:
  [U_bus] -> Bus Creator1/1  "U_bus"
  [I_abc] -> Bus Creator1/4  "I_abc"
  Bus Creator2/1 -> output/1
  [Sensor_Angle_e] -> Bus Creator4/1  "Sensor_Angle_e"
  [Sensor_Speed_m] -> Bus Creator4/2  "Sensor_Speed_m"
  Constant/1 -> Bus Creator1/3  "I_bus"
  Bus Creator1/1 -> Bus Creator2/1  "Elec_info"
  Bus Creator4/1 -> Bus Creator2/2  "Mach_info"
  [U_abc] -> Bus Creator1/2  "U_abc"
  [Q] -> Bus Creator6/4  "Q"
  [R] -> Bus Creator6/5  "R"
  [S] -> Bus Creator6/6  "S"
  [K] -> Bus Creator6/7  "K"
  [Err_code] -> Bus Creator2/4  "ErrCode"
  [E_alphabeta] -> Bus Creator6/1  "E_AlphaBeta"
  [Observer_Angle_e] -> Bus Creator6/2  "Observer_Angle_e"
  [Observer_Speed_m] -> Bus Creator6/3  "Observer_Speed_m"
  Bus Creator6/1 -> Bus Creator2/3  "Observer_info"

== system PMSM_FOC_sensorless/FOC/电流控制 ==
  note: 前馈加积分饱和补偿控制
  Idq* : Inport
  Speed~ : Inport  Port=2
  Vbus : Inport  Port=3
  Idq~ : Inport  Port=4
  Gain : Gain  Gain=(0.98-0.02)/sqrt(3)
  Gain1 : Gain  Gain=1/2
  Ki : Constant  Value=motor.Ls*20  OutDataTypeStr=single  SampleTime=-1
  Kp : Constant  Value=(motor.Ls/Ts)*0.2  OutDataTypeStr=single  SampleTime=-1
  Sum : Sum  Inputs=-+-
  Sum1 : Sum  Inputs=++|
  Sum2 : Sum  Inputs=+-|
  Sum3 : Sum  Inputs=|++
  前馈控制1 : Subsystem
  反馈控制 : slpidlib/PID Controller  Controller=PI  Form=Parallel  TimeDomain=Discrete-time  UseExternalTs=off  SampleTime=-1  IntegratorMethod=Forward Euler  FilterMethod=Forward Euler  ControllerParametersSource=external  P=1  I=1  UseKiTs=on  D=0  UseExternalDerivativeSource=off  N=100  UseFilter=on  TunerSelectOption=Transfer Function Based (PID Tuner App)  InitialConditionSource=internal  InitialConditionForIntegrator=0  InitialConditionForFilter=0  DifferentiatorICPrevScaledInput=0  ExternalReset=none  TrackingMode=off  Kt=1  LimitOutput=off  SatLimitsSource=internal  UpperSaturationLimit=drive.V_bus/2  LowerSaturationLimit=-drive.V_bus/2  LinearizeAsGain=on  AntiWindupMode=clamping  Kb=1  LimitIntegrator=off  UpperIntegratorSaturationLimit=inf  LowerIntegratorSaturationLimit=-inf  RndMeth=Simplest  POutMin=[]  POutMax=[]  IOutMin=[]  IOutMax=[]  DOutMin=[]  DOutMax=[]  NOutMin=[]  NOutMax=[]  SumOutMin=[]  SumOutMax=[]  SaturationOutDataTypeStr=Inherit: Inherit via back propagation  SaturationOutMin=[]  SaturationOutMax=[]  PParamMin=[]  PParamMax=[]  IParamMin=[]  IParamMax=[]  DParamMin=[]  DParamMax=[]  NParamMin=[]  NParamMax=[]  KbParamMin=[]  KbParamMax=[]  KtParamMin=[]  KtParamMax=[]  KbOutMin=[]  KbOutMax=[]  KtOutMin=[]  KtOutMax=[]  IntegratorOutMin=[]  IntegratorOutMax=[]  FilterOutMin=[]  FilterOutMax=[]  SumI1OutMin=[]  SumI1OutMax=[]  SumI2OutMin=[]  SumI2OutMax=[]  SumI3OutMin=[]  SumI3OutMax=[]  SumI4OutMin=[]  SumI4OutMax=[]  SumDOutMin=[]  SumDOutMax=[]  DifferentiatorOutMin=[]  DifferentiatorOutMax=[]  FilterDiffOutCoefMin=[]  FilterDiffOutCoefMax=[]  ReciprocalOutMin=[]  ReciprocalOutMax=[]  SumDenOutMin=[]  SumDenOutMax=[]  SumNumOutMin=[]  SumNumOutMax=[]  DivideOutMin=[]  DivideOutMax=[]  UdiffTsProdOutMin=[]  UdiffTsProdOutMax=[]  NTsProdOutMin=[]  NTsProdOutMax=[]  UintegralTsProdOutMin=[]  UintegralTsProdOutMax=[]  UngainTsProdOutMin=[]  UngainTsProdOutMax=[]  ClampingZeroOutDataTypeStr=Inherit: Inherit via back propagation  ClampingZeroOutMin=[]  ClampingZeroOutMax=[]  FilterDenConstantOutDataTypeStr=Inherit: Inherit via back propagation  FilterDenConstantOutMin=[]  FilterDenConstantOutMax=[]  PCopyOutDataTypeStr=Inherit: Inherit via back propagation  PCopyOutMin=[]  PCopyOutMax=[]  NCopyOutDataTypeStr=Inherit: Inherit via back propagation  NCopyOutMin=[]  NCopyOutMax=[]  IntegratorContinuousStateAttributes=''  IntegratorStateMustResolveToSignalObject=off  IntegratorRTWStateStorageClass=Auto  FilterContinuousStateAttributes=''  FilterStateMustResolveToSignalObject=off  FilterRTWStateStorageClass=Auto  ParallelPVariant=ExternalParameters  IdealPVariant=Disabled  IVariant=ExternalParameters  DVariant=Disabled  IntegratorVariant=Discrete  SatVariant=Disabled  AWVariant=Passthrough  PCopyVariant=Disabled  TRVariant=Disabled  FdbkBlocksVariant=Forward  IdealPFdbkVariant=Disabled  SatFdbkVariant=Disabled  DerivativeFilterVariant=Disabled  NVariant=Disabled  NCopyVariant=Disabled_SignalSpec  FilterICVariant=Disabled  IntegratorICVariant=InternalICs  ExternalResetVariant=Disabled  TRSumVariant=Passthrough  SumFdbkVariant=Disabled  SumVariant=Sum_PI  TsampFilterVariant=InternalTs  TsampNgainVariant=Passthrough  TsampIntegralVariant=Disabled_SignalSpec  ExternalSaturationOutDataTypeStr=Inherit: Same as second input  DerivativeSourceVariant=Disabled  PreIntVariant=InternalPreInt
  滞后补偿 : Delay
  滞后补偿1 : Delay  DelayLength=1
  滞后补偿2 : Delay  DelayLength=1
  电压限幅 : Subsystem
      settings: PortSchema="{\"entries\":[{\"content\":{\"sides\":[{\"content\":{\"connectorIds\":[\"In1\"]},\"type\":\"ConnectorPlacement.EquallySpacedRectSide\",\"uuid\":\"8318c52a-9d90-468d-b9ba-7dc43530864a\"},{\"content\":{\"connectorIds\":[\"Out1\"],\"side\":\"RIGHT\"},\"type\":\"ConnectorPlacement.EquallySpacedRectSide\",\"uuid\":\"ec35b037-8c54-4ea5-a44f-2157489f6ede\"},{\"content\":{\"connectorIds\":[\"In2\"],\"side\":\"TOP\"},\"type\":\"ConnectorPlacement.EquallySpacedRectSide\",\"uuid\":\"86589762-ebe7-4f54-bef4-fc17ac715e1b\"}]},\"type\":\"ConnectorPlacement.EquallySpacedConnector\",\"uuid\":\"5c9fe270-4db2-4b15-bc03-dab13b772a86\"}],\"packageUris\":[\"http://schema.mathworks.com/mf0/Connector/R2020b\"],\"version\":\"1.0\"}"
  非线性补偿 : Subsystem
  Udq* : Outport  VectorParamsAs1DForOutWhenUnconnected=off
  wires:
  反馈控制/1 -> Sum1/2  "反馈"
  Sum/1 -> 反馈控制/1  "ErrIdq"
  Idq~/1 -> 前馈控制1/3(IdqFb), Sum/1
  Ki/1 -> 反馈控制/3
  Kp/1 -> 反馈控制/2
  滞后补偿/1 -> Sum3/1, 滞后补偿2/1
  Vbus/1 -> Gain/1
  电压限幅/1(dq_out) -> Sum2/2, Udq*/1
  Speed~/1 -> 前馈控制1/1(ω)
  Gain/1 -> 电压限幅/2(Limit)
  Sum2/1 -> 非线性补偿/1(U_dq)  "Us_dq"
  非线性补偿/1(I_dq) -> 滞后补偿1/1
  滞后补偿2/1 -> Sum3/2
  Sum3/1 -> Gain1/1
  Gain1/1 -> Sum/2
  Sum1/1 -> Sum2/1, 电压限幅/1(dq_in)
  前馈控制1/1(FeedForward) -> Sum1/1  "前馈"
  Idq*/1 -> 滞后补偿/1, 前馈控制1/2(IdqRef)
  滞后补偿1/1 -> Sum/3

== system PMSM_FOC_sensorless/FOC/相电流计算 ==
  DIabc : Inport
  DA转换 : Gain  Gain=drive.ADC_Vref/(drive.ADC_MaxCount*2)  OutDataTypeStr=single
  Data Type Conversion : DataTypeConversion  OutDataTypeStr=single  SaturateOnIntegerOverflow=off  RndMeth=Floor
  Gain1 : Gain  Gain=1/3
  Sum : Sum  Inputs=|+-
  Sum of Elements : Sum  Inputs=+
  电流计算 : Gain  Gain=1/drive.I_gain
  Iabc : Outport
  wires:
  DA转换/1 -> 电流计算/1  "电压"
  DIabc/1 -> Data Type Conversion/1
  Data Type Conversion/1 -> DA转换/1
  Sum/1 -> Iabc/1
  Gain1/1 -> Sum/2
  Sum of Elements/1 -> Gain1/1
  电流计算/1 -> Sum/1, Sum of Elements/1

== system PMSM_FOC_sensorless/FOC/转速控制 ==
  Spd_ref : Inport
  Spd_fb : Inport  Port=2
  Constant : Constant  Value=0.015  OutDataTypeStr=single
  Constant1 : Constant  Value=0.2*Ts  OutDataTypeStr=single
  Constant3 : Constant  Value=0  OutDataTypeStr=single
  Math Function1 : Math  Operator=square
  Math Function2 : Math  Operator=square
  Math Function3 : Math  Operator=square
  PI控制器 : slpidlib/PID Controller  Controller=PI  Form=Parallel  TimeDomain=Discrete-time  UseExternalTs=off  SampleTime=Ts  IntegratorMethod=Forward Euler  FilterMethod=Forward Euler  ControllerParametersSource=external  P=1  I=1  UseKiTs=on  D=0  UseExternalDerivativeSource=off  N=100  UseFilter=on  TunerSelectOption=Transfer Function Based (PID Tuner App)  InitialConditionSource=external  InitialConditionForIntegrator=0  InitialConditionForFilter=0  DifferentiatorICPrevScaledInput=0  ExternalReset=level  TrackingMode=off  Kt=1  LimitOutput=on  SatLimitsSource=internal  UpperSaturationLimit=motor.T_rated  LowerSaturationLimit=-motor.T_rated  LinearizeAsGain=on  AntiWindupMode=clamping  Kb=1  LimitIntegrator=off  UpperIntegratorSaturationLimit=inf  LowerIntegratorSaturationLimit=-inf  RndMeth=Simplest  POutMin=[]  POutMax=[]  IOutMin=[]  IOutMax=[]  DOutMin=[]  DOutMax=[]  NOutMin=[]  NOutMax=[]  SumOutMin=[]  SumOutMax=[]  SaturationOutDataTypeStr=Inherit: Inherit via back propagation  SaturationOutMin=[]  SaturationOutMax=[]  PParamMin=[]  PParamMax=[]  IParamMin=[]  IParamMax=[]  DParamMin=[]  DParamMax=[]  NParamMin=[]  NParamMax=[]  KbParamMin=[]  KbParamMax=[]  KtParamMin=[]  KtParamMax=[]  KbOutMin=[]  KbOutMax=[]  KtOutMin=[]  KtOutMax=[]  IntegratorOutMin=[]  IntegratorOutMax=[]  FilterOutMin=[]  FilterOutMax=[]  SumI1OutMin=[]  SumI1OutMax=[]  SumI2OutMin=[]  SumI2OutMax=[]  SumI3OutMin=[]  SumI3OutMax=[]  SumI4OutMin=[]  SumI4OutMax=[]  SumDOutMin=[]  SumDOutMax=[]  DifferentiatorOutMin=[]  DifferentiatorOutMax=[]  FilterDiffOutCoefMin=[]  FilterDiffOutCoefMax=[]  ReciprocalOutMin=[]  ReciprocalOutMax=[]  SumDenOutMin=[]  SumDenOutMax=[]  SumNumOutMin=[]  SumNumOutMax=[]  DivideOutMin=[]  DivideOutMax=[]  UdiffTsProdOutMin=[]  UdiffTsProdOutMax=[]  NTsProdOutMin=[]  NTsProdOutMax=[]  UintegralTsProdOutMin=[]  UintegralTsProdOutMax=[]  UngainTsProdOutMin=[]  UngainTsProdOutMax=[]  ClampingZeroOutDataTypeStr=Inherit: Inherit via back propagation  ClampingZeroOutMin=[]  ClampingZeroOutMax=[]  FilterDenConstantOutDataTypeStr=Inherit: Inherit via back propagation  FilterDenConstantOutMin=[]  FilterDenConstantOutMax=[]  PCopyOutDataTypeStr=Inherit: Inherit via back propagation  PCopyOutMin=[]  PCopyOutMax=[]  NCopyOutDataTypeStr=Inherit: Inherit via back propagation  NCopyOutMin=[]  NCopyOutMax=[]  IntegratorContinuousStateAttributes=''  IntegratorStateMustResolveToSignalObject=off  IntegratorRTWStateStorageClass=Auto  FilterContinuousStateAttributes=''  FilterStateMustResolveToSignalObject=off  FilterRTWStateStorageClass=Auto  ParallelPVariant=ExternalParameters  IdealPVariant=Disabled  IVariant=ExternalParameters  DVariant=Disabled  IntegratorVariant=Discrete  SatVariant=Enabled  AWVariant=DiscClampingParallel  PCopyVariant=Disabled  TRVariant=Disabled  FdbkBlocksVariant=Forward  IdealPFdbkVariant=Disabled  SatFdbkVariant=Disabled  DerivativeFilterVariant=Disabled  NVariant=Disabled  NCopyVariant=Disabled_SignalSpec  FilterICVariant=Disabled  IntegratorICVariant=ExternalICs  ExternalResetVariant=ExternalReset  TRSumVariant=Passthrough  SumFdbkVariant=Disabled  SumVariant=Sum_PI  TsampFilterVariant=InternalTs  TsampNgainVariant=Passthrough  TsampIntegralVariant=Disabled_SignalSpec  ExternalSaturationOutDataTypeStr=Inherit: Same as second input  DerivativeSourceVariant=Disabled  PreIntVariant=InternalPreInt
  Saturation1 : Saturate  UpperLimit=motor.radps_max  LowerLimit=-motor.radps_max
  Sum : Sum  Inputs=|+-
  Sum1 : Sum  Inputs=++|
  判断 : RelationalOperator  Operator=<  OutDataTypeStr=boolean  RndMeth=Simplest  InputSameDT=off
  额定转速2% : Constant  Value=motor.radps_rated*0.00  OutDataTypeStr=single
  Torque* : Outport
  wires:
  Constant/1 -> PI控制器/2
  PI控制器/1 -> Torque*/1  "扭矩"
  Sum/1 -> PI控制器/1
  Spd_fb/1 -> Math Function2/1, Sum/2
  Spd_ref/1 -> Saturation1/1
  Constant1/1 -> PI控制器/3
  Saturation1/1 -> Math Function1/1, Sum/1
  Math Function2/1 -> Sum1/2
  Math Function1/1 -> Sum1/1
  Sum1/1 -> 判断/1
  判断/1 -> PI控制器/4
  额定转速2%/1 -> Math Function3/1
  Constant3/1 -> PI控制器/5
  Math Function3/1 -> 判断/2

== system PMSM_FOC_sensorless/Inverter/AD转换 ==
  analog : Inport
  Gain1 : Gain  Gain=drive.ADC_MaxCount/drive.ADC_Vref  OutDataTypeStr=int16
  Sum : Sum  Inputs=|++
  Unit Delay : UnitDelay  SampleTime=-1
  digital : Outport
  wires:
  Gain1/1 -> Unit Delay/1, Sum/1
  analog/1 -> Gain1/1
  Sum/1 -> digital/1
  Unit Delay/1 -> Sum/2

== system PMSM_FOC_sensorless/Inverter/模拟MOS管截至状态 ==
  Iabc : Inport
  Constant : Constant  Value=0.5  OutDataTypeStr=single
  Gain2 : Gain  Gain=-0.1  OutDataTypeStr=single
  Saturation : Saturate  UpperLimit=1  LowerLimit=0
  Sum : Sum  Inputs=|++
  Out1 : Outport
  wires:
  Iabc/1 -> Gain2/1
  Saturation/1 -> Out1/1
  Constant/1 -> Sum/2
  Gain2/1 -> Sum/1
  Sum/1 -> Saturation/1

== system PMSM_FOC_sensorless/Inverter/正常PWM调制 ==
  note: 添加死区
  Dabc : Inport
  Iabc : Inport  Port=2
  Gain2 : Gain  Gain=(drive.dead_time*drive.f_PWM)  OutDataTypeStr=single
  Gain3 : Gain  Gain=1/drive.CNT_PWM  OutDataTypeStr=single
  Sign : Signum
  Sum : Sum  Inputs=-+|
  Unit Delay : UnitDelay  SampleTime=-1
  Out1 : Outport
  wires:
  Unit Delay/1 -> Gain3/1
  Gain3/1 -> Sum/2
  Iabc/1 -> Sign/1
  Dabc/1 -> Unit Delay/1
  Sign/1 -> Gain2/1
  Gain2/1 -> Sum/1
  Sum/1 -> Out1/1

== system PMSM_FOC_sensorless/Inverter/母线压降 ==
  VCC : Inport
  P : Inport  Port=2
  Divide4 : Product  Inputs=*/
  Gain : Gain  Gain=drive.R_bus
  Saturation : Saturate  UpperLimit=48  LowerLimit=12
  Sum : Sum  Inputs=|+-
  Unit Delay : UnitDelay  SampleTime=-1
  U_bus : Outport
  wires:
  Sum/1 -> Unit Delay/1, U_bus/1
  VCC/1 -> Sum/1
  P/1 -> Divide4/1
  Divide4/1 -> Gain/1
  Gain/1 -> Sum/2
  Saturation/1 -> Divide4/2
  Unit Delay/1 -> Saturation/1

== system PMSM_FOC_sensorless/Inverter/母线电压采样 ==
  note: 待增加噪声和滞后环节
  U_bus : Inport
  Sum : Sum  Inputs=|++
  Unit Delay : UnitDelay  SampleTime=-1
  电压采样 : Gain  Gain=(drive.V_gain*drive.ADC_MaxCount)/drive.ADC_Vref  OutDataTypeStr=int16
  AD_Ubus : Outport
  wires:
  电压采样/1 -> Unit Delay/1, Sum/1
  Unit Delay/1 -> Sum/2
  Sum/1 -> AD_Ubus/1
  U_bus/1 -> 电压采样/1

== system PMSM_FOC_sensorless/Inverter/采样芯片 ==
  Iabc : Inport
  Saturation : Saturate  UpperLimit=drive.ADC_Vref*0.9  LowerLimit=drive.ADC_Vref*0.1
  Sum : Sum  Inputs=|++  OutDataTypeStr=single  AccumDataTypeStr=single
  偏置&噪声 : RandomNumber  Mean=drive.I_offset  Variance=drive.I_noise.^2  Seed=[1,2,3]  SampleTime=Ts
  电流采样增益 : Gain  Gain=drive.I_gain  OutDataTypeStr=single
  Isabc : Outport
  wires:
  电流采样增益/1 -> Sum/1
  Sum/1 -> Saturation/1
  偏置&噪声/1 -> Sum/2  "电压噪声"
  Iabc/1 -> 电流采样增益/1
  Saturation/1 -> Isabc/1

== system PMSM_FOC_sensorless/PMSM/Subsystem2 ==
  0-2pi : Inport
  Constant3 : Constant  Value=-pi  OutDataTypeStr=single
  Constant4 : Constant  Value=pi  OutDataTypeStr=single
  Gain6 : Gain  Gain=-2*pi  OutDataTypeStr=single
  Gain7 : Gain  Gain=2*pi  OutDataTypeStr=single
  Relational Operator2 : RelationalOperator  Operator=<  RndMeth=Simplest  InputSameDT=off
  Relational Operator3 : RelationalOperator  Operator=<  RndMeth=Simplest  InputSameDT=off
  Sum3 : Sum  Inputs=+++
  -pi-pi : Outport
  wires:
  Sum3/1 -> -pi-pi/1
  Gain7/1 -> Sum3/3
  Gain6/1 -> Sum3/1
  Relational Operator3/1 -> Gain6/1
  Relational Operator2/1 -> Gain7/1
  0-2pi/1 -> Relational Operator3/2, Sum3/2, Relational Operator2/1
  Constant3/1 -> Relational Operator2/2
  Constant4/1 -> Relational Operator3/1

== system PMSM_FOC_sensorless/数据可视化/angle limit2 ==
  In : Inport
  Constant2 : Constant  Value=-pi  OutDataTypeStr=single
  Constant4 : Constant  Value=pi  OutDataTypeStr=single
  Gain6 : Gain  Gain=-2*pi  OutDataTypeStr=single
  Gain7 : Gain  Gain=2*pi  OutDataTypeStr=single
  Relational Operator2 : RelationalOperator  Operator=<  RndMeth=Simplest  InputSameDT=off
  Relational Operator3 : RelationalOperator  Operator=<  RndMeth=Simplest  InputSameDT=off
  Sum3 : Sum  Inputs=+++
  Out : Outport
  wires:
  Constant2/1 -> Relational Operator2/2
  In/1 -> Relational Operator3/2, Sum3/2, Relational Operator2/1
  Constant4/1 -> Relational Operator3/1
  Relational Operator3/1 -> Gain6/1
  Gain7/1 -> Sum3/3
  Relational Operator2/1 -> Gain7/1
  Gain6/1 -> Sum3/1
  Sum3/1 -> Out/1
